simulink model "HQ"  (R2018a)
settings: Solver=VariableStepAuto  StartTime=0.0  StopTime=10.0  MaxStep=0.01  RelTol=1e-3
InitFcn:
  | var_HQ
values from neighbouring files (symbols this model uses):
  lev_max = 1000    [fcn.m]    (also in var_HQ.m)
  rou = 0.9    [fcn.m]    (also in var_HQ.m)
  u_min = 0.02    [fcn.m]    (also in var_HQ.m)
settings Model: Creator=Administrator  LastModifiedBy=Administrator

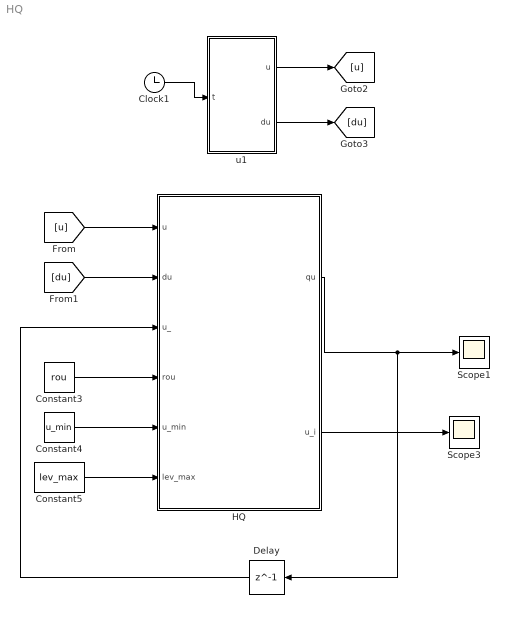
== system HQ ==
  Clock1 : Clock
  Constant3 : Constant  Value=rou
  Constant4 : Constant  Value=u_min
  Constant5 : Constant  Value=lev_max
  Delay : Delay  DelayLength=1  InitialCondition=0
  HQ : MATLAB Function  TreatAsAtomicUnit=on
  Scope1 : Scope
  Scope3 : Scope
  u1 : MATLAB Function  TreatAsAtomicUnit=on
  wires:
  HQ/1(qu) -> Delay/1, Scope1/1
  u1/1(u) -> [u]
  Clock1/1 -> u1/1(t)
  [u] -> HQ/1(u)
  Constant5/1 -> HQ/6(lev_max)
  Constant4/1 -> HQ/5(u_min)
  Constant3/1 -> HQ/4(rou)
  u1/2(du) -> [du]
  [du] -> HQ/2(du)
  Delay/1 -> HQ/3(u_)
  HQ/2(u_i) -> Scope3/1

== matlab function HQ/HQ ==
  data: qu output; u input; du input; u_ input; rou input; u_min input; lev_max input; u_i output
function [qu,u_i]  = fcn(u,du,u_,rou,u_min,lev_max)
ii=1:lev_max;
ind=zeros(length(1:lev_max),3);
delta=(1-rou)/(1+rou);
ind(ii,1)=(rou.^(1-ii)).*u_min;
ind(ii,2)=ind(ii,1)./(1-delta);
ind(ii,3)=(ind(ii,1).*(1+delta))./(1-delta);
flag=sign(du);
qu=3;
u_i=-1;
switch flag
    case -1
        u_i=Find_U_I(u,ind,-1);
        if (abs(u) > (u_i/(1+delta)))&&(abs(u) <= u_i)
            qu=u_i*sign(u);
        elseif (abs(u) > u_i)&&(abs(u) <= u_i/(1-delta))
            qu=u_i*(1+delta)*sign(u);
        elseif (abs(u) >= 0)&&(abs(u) < u_min/(1+delta))
            qu=0;
        end
    case 1
        u_i=Find_U_I(u,ind,1);
        if (abs(u) > u_i)&&(abs(u) <= u_i/(1-delta))
            qu=u_i*sign(u);
        elseif (abs(u) > u_i/(1-delta))&&(abs(u) <= u_i*(1+delta)/(1-delta))
            qu=u_i*(1+delta)*sign(u);
%         elseif (abs(u) >= u_min/(1+delta))&&(abs(u) <= u_min)
%             qu=0;
%             break;
        elseif (abs(u) >= 0)&&(abs(u) <= u_min)
            qu=0;
        end
    case 0
        qu=u_;
end

== matlab function HQ/u1 ==
  data: t input; u output; du output
function [u,du]   = fcn(t)
% function u    = fcn(t)
u=sin(t);
du=cos(t);
